simulink model "APF_SoftLanding_Quadrotor"  (R2023a)
settings: Solver=VariableStepAuto  StartTime=0.0  StopTime=120  RelTol=1e-3
values from neighbouring files (symbols this model uses):
  alpha_t = pi/2    (= 1.57079632679)    [Parameters.m]
  d0 = 7    [Parameters.m]
  k1 = 0.1395    [Parameters.m]
  k2 = 0.1784    [Parameters.m]
  k3 = 0.0442    [Parameters.m]
  ka = 0.2    [Parameters.m]
  katt = 10    [Parameters.m]
  kb = 0.6    [Parameters.m]
  kc = 0.4    [Parameters.m]
  krep = 90000    [Parameters.m]
  m = 5    [Parameters.m]
  maxRange = 10    [Parameters.m]
  n = 3    [Parameters.m]
  P_psi_lead = 2    [Parameters.m]
  P_vel_lead = 5    [Parameters.m]
  posHpad = [-25 -25 0]    [Parameters.m]
  Rmin = 0.1    [Parameters.m]
  target = [-25 -25 -5]    [Parameters.m]
  theta_des = pi/4    (= 0.785398163397)    [Parameters.m]
  thresholdLanding = 15    [Parameters.m]
  v_max = 2    [Parameters.m]
  zeta_des = 0    [Parameters.m]
  zGround = -0.15    [Parameters.m]
undefined symbols (not defined in the file or in its folder): Lidar, numobs, obs, platformUAV
libraries: uavsimlib x5, sharedtransform x2, uavalgslib x1, uavutilslib x1
(part 1 of 3)

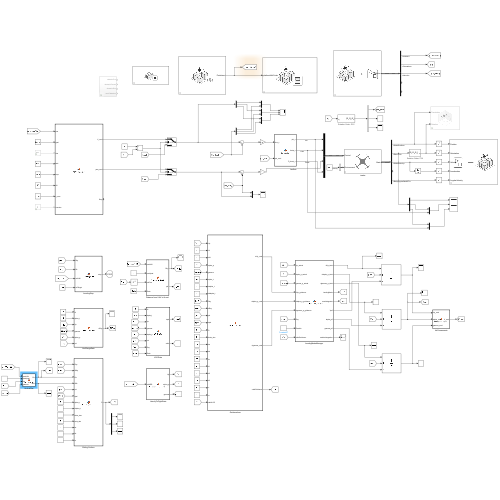
[thumbnail: Simulink's stored preview of the top-level diagram]
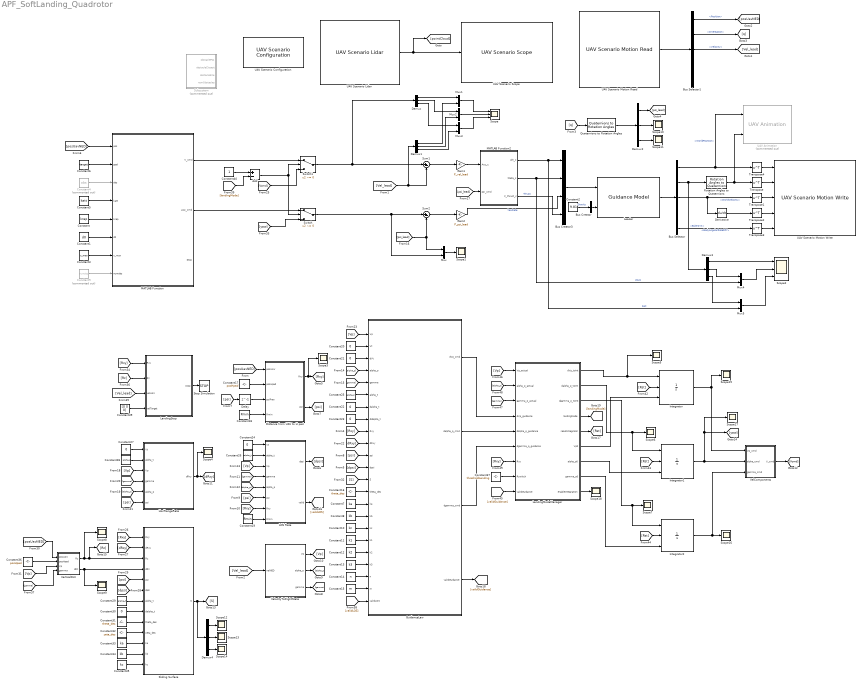
== system APF_SoftLanding_Quadrotor ==
  Add : Sum  Inputs=+-
  Bus Creator : BusCreator  Inputs=1  OutDataTypeStr=Bus: MultirotorGuidanceEnvironmentBus  NonVirtualBus=on
  Bus Creator3 : BusCreator  Inputs=4  OutDataTypeStr=Bus: MultirotorGuidanceControlBus  NonVirtualBus=on
  Bus Selector : BusSelector  OutputSignals=WorldPosition,EulerZYX,WorldVelocity,Thrust,BodyAngularRateRPY
  Bus Selector1 : BusSelector  OutputSignals=Position,Orientation,Velocity,Acceleration,AngularVelocity
  Constant : Constant  Value=krep
  Constant1 : Constant  Value=d0
  Constant10 : Constant  Value=kc
  Constant11 : Constant  Value=k1
  Constant12 : Constant  Value=k2
  Constant13 : Constant  Value=k3
  Constant14 : Constant  Value=n
  Constant15 : Constant  Value=m
  Constant16 : Constant  Value=theta_des
  Constant17 : Constant  Value=posHpad
  Constant18 : Constant  Value=Rmin
  Constant19 : Constant  Value=Rmin
  Constant2 : Constant  Value=9.81
  Constant{20..24,27,30} (7 alike) : Constant  Value=0
  Constant{25..26,28..29} (4 alike) : Constant  Value=alpha_t
  Constant3 : Constant  Value=v_max
  Constant31 : Constant  Value=theta_des
  Constant32 : Constant  Value=zeta_des
  Constant33 : Constant  Value=ka
  Constant34 : Constant  Value=kb
  Constant35 : Constant  Value=kc
  Constant36 : Constant  Value=posHpad
  Constant37 : Constant  Value=thresholdLanding
  Constant39 : Constant  Value=[0 0 0]
  Constant4 : Constant  Commented=on  Value=obs  VectorParams1D=off
  Constant40 : Constant
  Constant5 : Constant  Value=katt
  Constant6 : Constant  Value=target
  Constant7 : Constant  Value=ka
  Constant8 : Constant  Value=kb
  Constant9 : Constant  Commented=on  Value=numobs
  Delay : Delay  DelayLength=1
  Demux{,1..4} (5 alike) : Demux  Outputs=3
  Derivative : Derivative
  "Distance from UAV to H pad " : MATLAB Function  TreatAsAtomicUnit=on
  Gain1 : Gain  Gain=P_vel_lead
  Gain2 : Gain  Gain=P_psi_lead
  GuidanceLaw : MATLAB Function  TreatAsAtomicUnit=on
  HoriRangeRate : MATLAB Function  TreatAsAtomicUnit=on
  Integrator : Integrator  ExternalReset=rising  InitialConditionSource=external  InitialCondition=0.001
  Integrator1 : Integrator  ExternalReset=rising  InitialConditionSource=external
  Integrator2 : Integrator  ExternalReset=rising  InitialConditionSource=external
  LOS Rate : MATLAB Function  TreatAsAtomicUnit=on
  LandingModeManager : MATLAB Function  TreatAsAtomicUnit=on
  LandingStop : MATLAB Function  TreatAsAtomicUnit=on
  Leader : uavalgslib/Guidance Model  ModelType=MultirotorGuidance  SpecifiedDataType=double  SimulateUsing=Interpreted execution  InitialWorldPositionMultirotor=[-50; -50; -5]  InitialWorldVelocityMultirotor=[0.01; 0.01; 0.01]  InitialEulerZYXMultirotor=[0; 0; 0]  InitialBodyAngularRateRPYMultirotor=[0; 0; 0]  InitialThrustMultirotor=0  InitialNorthFixedWing=0  InitialEastFixedWing=0  InitialHeightFixedWing=0  InitialAirSpeedFixedWing=0  InitialHeadingAngleFixedWing=0  InitialFlightPathAngleFixedWing=0  InitialRollAngleFixedWing=0  InitialRollAngleRateFixedWing=0  PDRollMultirotor=[3402.97,116.67]  PDPitchMultirotor=[3402.97, 116.67]  PYawRateMultirotor=1950  PThrustMultirotor=3900  MassMultirotor=0.1  PHeightFixedWing=3.9  PHeadingAngleFixedWing=3.9  PFlightPathAngleFixedWing=39  PDRollFixedWing=[3402.97, 116.67]  PAirSpeedFixedWing=1  FlightPathAngleLimitsFixedWing=[-pi/2, pi/2]  StateBusName='MultirotorGuidanceStateBus'  ControlBusName='MultirotorGuidanceControlBus'  EnvironmentBusName='MultirotorGuidanceEnvironmentBus'  DataType=double
  MATLAB Function : MATLAB Function  TreatAsAtomicUnit=on
  MATLAB Function2 : MATLAB Function  TreatAsAtomicUnit=on
  Mux{,1..5} (6 alike) : Mux  Inputs=2
  Quaternions to Rotation Angles : sharedtransform/Quaternions to Rotation Angles  rotationOrder=ZYX  aMode=aMode
  Rotation Angles to Quaternions : sharedtransform/Rotation Angles to Quaternions  rotationOrder=ZYX  aMode=aMode
  Scope : Scope  NumInputPorts=3
  Scope{1,3..18} (17 alike) : Scope
  Scope2 : Scope  NumInputPorts=3
  Sliding Surface : MATLAB Function  TreatAsAtomicUnit=on
  Stop Simulation : Stop
  Subsystem : Subsystem  Commented=on
  Sum1 : Sum  Inputs=|+-
  Sum2 : Sum  Inputs=|+-
  Switch : Switch  Criteria=u2 ~= 0  Threshold=thresholdLanding  SaturateOnIntegerOverflow=off  InputSameDT=off
  Switch1 : Switch  Criteria=u2 ~= 0  Threshold=thresholdLanding  SaturateOnIntegerOverflow=off  InputSameDT=off
  Transpose{,1..4} (5 alike) : Math  Operator=transpose
  UAV Animation : uavutilslib/UAV Animation  Commented=on  UAVType=Multirotor  UAVSize=1  InertialZDirection=Down  SampleTime=-1
  UAV Scenario Configuration : uavsimlib/UAV Scenario Configuration  Priority=-1  UAVScenarioObject=sceneUAV  SampleTime=0.1  UpdateParam=false  SensorMotionBusName='SensorMotionBus'  PlatformMotionBusName='PlatformMotionBus'  ScenarioMotionBusName='ScenarioMotionBus'  ScenarioMotionSignalName='ScenarioMotions'
  UAV Scenario Lidar : uavsimlib/UAV Scenario Lidar  Priority=1  SensorName=platformUAV/Lidar  MaxRange=10  RangeAccuracy=0.002  AzimuthLimits=[ -43.5, 43.5 ]  AzimuthResolution=0.16  ElevationLimits=[ -29, 29 ]  ElevationResolution=1.25  HasNoise=on  HasOrganizedOutput=off  SampleTime=0.1
  UAV Scenario Motion Read : uavsimlib/UAV Scenario Motion Read  Priority=1  EntityName='platformUAV'  ReferenceFrame=NED
  UAV Scenario Motion Write : uavsimlib/UAV Scenario Motion Write  Priority=0  PlatName='platformUAV'  ReferenceFrame=NED
  UAV Scenario Scope : uavsimlib/UAV Scenario Scope  Priority=1  SensorNameTable={ 'platformUAV/Lidar', 'on' }  SampleTime=0.1
  VelComponents : MATLAB Function  TreatAsAtomicUnit=on
  VelocityToFlightState : MATLAB Function  TreatAsAtomicUnit=on
  VerticalDist : MATLAB Function  TreatAsAtomicUnit=on
  wires:
  Bus Creator/1 -> Leader/2
  Constant2/1 -> Bus Creator/1  "Gravity"
  Leader/1 -> Bus Selector/1
  Demux2/1 -> [psi_lead]
  Gain1/1 -> MATLAB Function2/1(Acc_c)
  Bus Creator3/1 -> Leader/1
  MATLAB Function2/1(phi_c) -> Mux5/2, Bus Creator3/1  "Roll"
  MATLAB Function2/2(theta_c) -> Mux4/2, Bus Creator3/2  "Pitch"
  Sum1/1 -> Gain1/1
  Sum2/1 -> Gain2/1
  [psi_lead] -> MATLAB Function2/2(psi_cmd)
  Gain2/1 -> Bus Creator3/3  "YawRate"
  MATLAB Function2/3(F_thrust_c) -> Bus Creator3/4  "Thrust"
  Bus Selector/1 -> Transpose4/1, UAV Animation/1  "<WorldPosition>"
  [Vel_lead] -> Demux1/1, Sum1/2
  UAV Scenario Lidar/1 -> [pointCloud], UAV Scenario Scope/1
  Bus Selector/2 -> Rotation Angles to Quaternions/1, Demux3/1  "<EulerZYX>"
  Rotation Angles to Quaternions/1 -> Transpose/1, UAV Animation/2
  Bus Selector/3 -> Transpose1/1, Derivative/1  "<WorldVelocity>"
  UAV Scenario Motion Read/1 -> Bus Selector1/1
  Quaternions to Rotation Angles/1 -> Demux2/1
  Bus Selector1/3 -> [Vel_lead]  "<Velocity>"
  Bus Selector1/1 -> [posUavNED]  "<Position>"
  Bus Selector1/2 -> [q]  "<Orientation>"
  [q] -> Quaternions to Rotation Angles/1
  [posUavNED] -> MATLAB Function/1(pos)
  Transpose4/1 -> UAV Scenario Motion Write/1
  Transpose/1 -> UAV Scenario Motion Write/2
  Transpose1/1 -> UAV Scenario Motion Write/3
  Derivative/1 -> Transpose2/1
  Transpose2/1 -> UAV Scenario Motion Write/4
  Bus Selector/5 -> Transpose3/1  "<BodyAngularRateRPY>"
  Transpose3/1 -> UAV Scenario Motion Write/5
  Mux/1 -> Scope1/1
  [psi_lead] -> Mux/1, Sum2/2
  Mux1/1 -> Scope/1
  Demux/1 -> Mux1/1
  Demux1/1 -> Mux1/2
  Mux2/1 -> Scope/2
  Demux/2 -> Mux2/1
  Demux1/2 -> Mux2/2
  Mux3/1 -> Scope/3
  Demux1/3 -> Mux3/2
  Demux/3 -> Mux3/1
  Constant4/1 -> MATLAB Function/3(obs)
  Constant9/1 -> MATLAB Function/8(numobs)
  Demux3/1 -> Scope2/1
  Mux4/1 -> Scope2/2
  Demux3/2 -> Mux4/1
  Mux5/1 -> Scope2/3
  Demux3/3 -> Mux5/1
  Constant5/1 -> MATLAB Function/4(katt)
  Constant/1 -> MATLAB Function/5(krep)
  Constant1/1 -> MATLAB Function/6(d0)
  Constant3/1 -> MATLAB Function/7(v_max)
  Constant11/1 -> GuidanceLaw/18(k1)
  Constant13/1 -> GuidanceLaw/20(k3)
  Constant14/1 -> GuidanceLaw/21(n)
  Constant15/1 -> GuidanceLaw/22(m)
  Constant7/1 -> GuidanceLaw/15(ka)
  Constant8/1 -> GuidanceLaw/16(kb)
  Constant10/1 -> GuidanceLaw/17(kc)
  Constant12/1 -> GuidanceLaw/19(k2)
  Constant16/1 -> GuidanceLaw/14(theta_des)
  Constant17/1 -> "Distance from UAV to H pad "/2(posHpad)
  [posUavNED] -> "Distance from UAV to H pad "/1(posUAV)
  Delay/1 -> "Distance from UAV to H pad "/3(psiPrev)
  "Distance from UAV to H pad "/1(Rxy) -> Scope3/1, [Rxy]
  [Rxy] -> GuidanceLaw/9(Rxy)
  Constant18/1 -> "Distance from UAV to H pad "/4(Rmin)
  Constant19/1 -> LOS Rate/8(Rmin)
  Constant20/1 -> GuidanceLaw/2(Vt)
  Constant21/1 -> GuidanceLaw/3(dVt)
  Constant23/1 -> GuidanceLaw/8(ddalpha_t)
  Constant22/1 -> GuidanceLaw/7(dalpha_t)
  [Vel_lead] -> VelocityToFlightState/1(velNED)
  LOS Rate/1(dpsi) -> [dpsi]
  [dpsi] -> GuidanceLaw/12(dpsi)
  "Distance from UAV to H pad "/2(psi) -> [psi]
  [psi] -> Delay/1
  [psi] -> GuidanceLaw/11(psi)
  [psi] -> LOS Rate/6(psi)
  [Rxy] -> LOS Rate/7(Rxy)
  Constant24/1 -> LOS Rate/1(Vt)
  Constant25/1 -> GuidanceLaw/6(alpha_t)
  VelocityToFlightState/3(gamma) -> [gamma]
  [gamma] -> LOS Rate/4(gamma)
  VelocityToFlightState/2(alpha_p) -> [alpha_p]
  [alpha_p] -> LOS Rate/5(alpha_p)
  VelocityToFlightState/1(Vp) -> [Vp]
  [Vp] -> LOS Rate/3(Vp)
  Constant26/1 -> LOS Rate/2(alpha_t)
  [alpha_p] -> GuidanceLaw/4(alpha_p)
  [gamma] -> GuidanceLaw/5(gamma)
  HoriRangeRate/1(dRxy) -> Scope4/1, [dRxy]
  [Vp] -> HoriRangeRate/3(Vp)
  [alpha_p] -> HoriRangeRate/5(alpha_p)
  [gamma] -> HoriRangeRate/4(gamma)
  [psi] -> HoriRangeRate/6(psi)
  [dRxy] -> GuidanceLaw/10(dRxy)
  Constant6/1 -> MATLAB Function/2(goal)
  Switch1/1 -> Demux/1, Sum1/1
  MATLAB Function/1(V_cmd) -> Switch1/1
  Switch/1 -> Mux/2, Sum2/1
  MATLAB Function/2(yaw_cmd) -> Switch/1
  GuidanceLaw/1(dVp_cmd) -> LandingModeManager/4(dVp_guidance)
  GuidanceLaw/2(dalpha_p_cmd) -> LandingModeManager/5(dalpha_p_guidance)
  GuidanceLaw/3(dgamma_cmd) -> LandingModeManager/6(dgamma_p_guidance)
  [Vp] -> GuidanceLaw/1(Vp)
  Constant27/1 -> HoriRangeRate/1(Vt)
  Constant28/1 -> HoriRangeRate/2(alpha_t)
  Sliding Surface/1(S) -> Demux4/1, [S]
  [Rxy] -> Sliding Surface/1(Rxy)
  [dRxy] -> Sliding Surface/2(dRxy)
  [psi] -> Sliding Surface/5(psi)
  [dpsi] -> Sliding Surface/6(dpsi)
  VerticalDist/2(dRz) -> Scope9/1, Sliding Surface/4(dRz)
  VerticalDist/1(Rz) -> Sliding Surface/3(Rz), [Rz], Scope8/1
  [posUavNED] -> VerticalDist/1(posUAV)
  Constant29/1 -> Sliding Surface/7(alpha_t)
  Constant30/1 -> Sliding Surface/8(dalpha_t)
  Constant31/1 -> Sliding Surface/9(theta_des)
  Constant32/1 -> Sliding Surface/10(zeta_des)
  Constant34/1 -> Sliding Surface/12(kb)
  Constant33/1 -> Sliding Surface/11(ka)
  Constant35/1 -> Sliding Surface/13(kc)
  Constant36/1 -> VerticalDist/2(posHpad)
  [S] -> GuidanceLaw/13(S)
  [Vcmd] -> Switch1/3
  [yaw] -> Switch/3
  LandingStop/1(stop) -> Stop Simulation/1
  [Rxy] -> LandingStop/1(Rxy)
  [Rz] -> LandingStop/2(Rz)
  [Vel_lead] -> LandingStop/3(velUAV)
  Constant39/1 -> LandingStop/4(velTarget)
  [Vp] -> VerticalDist/3(Vp)
  [gamma] -> VerticalDist/4(gamma)
  Demux2/2 -> Scope10/1
  Demux2/3 -> Scope11/1
  Demux4/1 -> Scope12/1
  Demux4/2 -> Scope13/1
  Demux4/3 -> Scope14/1
  LOS Rate/2(valid) -> [validLOS]
  [validLOS] -> GuidanceLaw/23(validLOS)
  GuidanceLaw/4(validGuidance) -> [validGuidance]
  [validGuidance] -> LandingModeManager/9(validGuidance)
  [Rst] -> Integrator1/2
  [Rst] -> Integrator/2
  [Rst] -> Integrator2/2
  LandingModeManager/1(dVp_toInt) -> Scope5/1, Integrator/1
  Integrator/1 -> Scope15/1, VelComponents/1(Vp_cmd)
  Integrator1/1 -> Scope17/1, [yaw], VelComponents/2(alpha_cmd)
  VelComponents/1(V_cmd) -> [Vcmd]
  Integrator2/1 -> VelComponents/3(gamma_cmd), Scope16/1
  LandingModeManager/2(dalpha_p_toInt) -> Integrator1/1, Scope6/1
  LandingModeManager/3(dgamma_p_toInt) -> Integrator2/1, Scope7/1
  LandingModeManager/5(resetIntegrator) -> [Rst]
  [Vp] -> LandingModeManager/1(Vp_actual)
  [gamma] -> LandingModeManager/3(gamma_p_actual)
  [alpha_p] -> LandingModeManager/2(alpha_p_actual)
  [Rxy] -> LandingModeManager/7(Rxy)
  Constant37/1 -> LandingModeManager/8(Rswitch)
  LandingModeManager/6(Vp0) -> Integrator/3
  LandingModeManager/7(alpha_p0) -> Integrator1/3
  LandingModeManager/8(gamma_p0) -> Integrator2/3
  LandingModeManager/9(enableIntegration) -> Scope18/1
  LandingModeManager/4(landingMode) -> [landingMode]
  [landingMode] -> Add/2
  Add/1 -> Switch1/2, Switch/2
  Constant40/1 -> Add/1

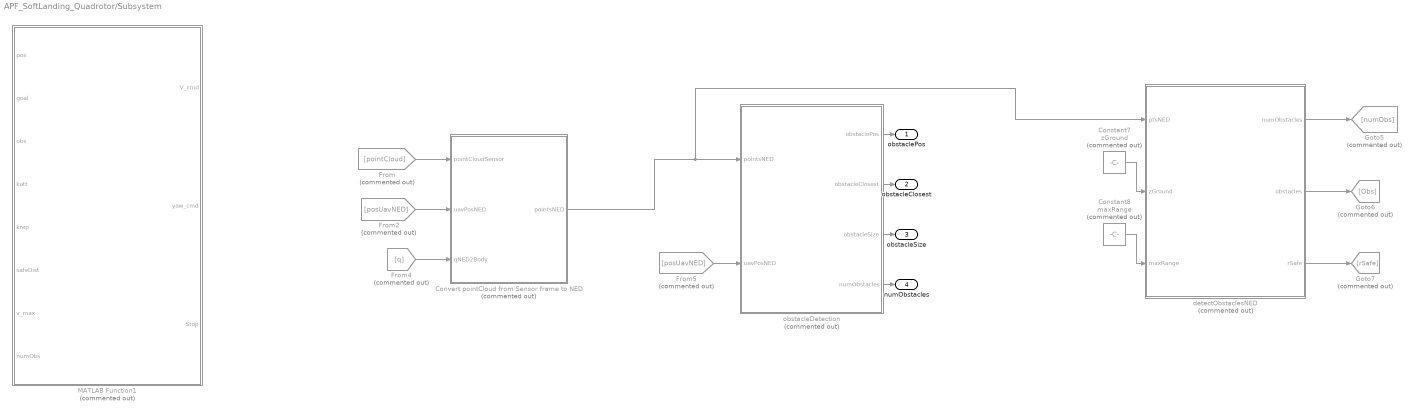
== system APF_SoftLanding_Quadrotor/Subsystem ==
  Constant7 : Constant  Commented=on  Value=zGround
  Constant8 : Constant  Commented=on  Value=maxRange
  Convert pointCloud from Sensor frame to NED : MATLAB Function  Commented=on  TreatAsAtomicUnit=on
  From : From  Commented=on  GotoTag=pointCloud
  From2 : From  Commented=on  GotoTag=posUavNED
  From4 : From  Commented=on  GotoTag=q
  From5 : From  Commented=on  GotoTag=posUavNED
  Goto5 : Goto  Commented=on  GotoTag=numObs
  Goto6 : Goto  Commented=on  GotoTag=Obs
  Goto7 : Goto  Commented=on  GotoTag=rSafe
  MATLAB Function1 : MATLAB Function  Commented=on  TreatAsAtomicUnit=on
  detectObstaclesNED : MATLAB Function  Commented=on  TreatAsAtomicUnit=on
  obstacleDetection : MATLAB Function  Commented=on  TreatAsAtomicUnit=on
  obstaclePos : Outport
  obstacleClosest : Outport  Port=2
  obstacleSize : Outport  Port=3
  numObstacles : Outport  Port=4
  wires:
  From4/1 -> Convert pointCloud from Sensor frame to NED/3(qNED2Body)
  Convert pointCloud from Sensor frame to NED/1(pointsNED) -> detectObstaclesNED/1(ptsNED), obstacleDetection/1(pointsNED)
  From2/1 -> Convert pointCloud from Sensor frame to NED/2(uavPosNED)
  detectObstaclesNED/1(numObstacles) -> Goto5/1
  obstacleDetection/1(obstaclePos) -> obstaclePos/1
  From/1 -> Convert pointCloud from Sensor frame to NED/1(pointCloudSensor)
  detectObstaclesNED/2(obstacles) -> Goto6/1
  Constant8/1 -> detectObstaclesNED/3(maxRange)
  Constant7/1 -> detectObstaclesNED/2(zGround)
  detectObstaclesNED/3(rSafe) -> Goto7/1
  From5/1 -> obstacleDetection/2(uavPosNED)
  obstacleDetection/3(obstacleSize) -> obstacleSize/1
  obstacleDetection/2(obstacleClosest) -> obstacleClosest/1
  obstacleDetection/4(numObstacles) -> numObstacles/1

== matlab function APF_SoftLanding_Quadrotor/MATLAB Function2 ==
function [phi_c, theta_c, F_thrust_c] = Conversion(Acc_c, psi_cmd)

% =========================================================
% Nonlinear acceleration -> attitude/thrust conversion
% Coordinate frame: NED
%
% Acc_c   = [aN; aE; aD] [m/s^2]
% psi_cmd = desired yaw  [rad]
% =========================================================

g = 9.81;
m = 0.1;     % kg

aN = Acc_c(1);
aE = Acc_c(2);
aD = Acc_c(3);

psi = psi_cmd;

% ---------------------------------------------------------
% Required thrust vector
%
% m*a = m*g*e3 - T*b3
%
% Therefore:
%
% T*b3 = m*[ -aN, -aE, g-aD ]
% ---------------------------------------------------------

fN = -aN;
fE = -aE;
fD =  g - aD;

f_norm = sqrt(fN^2 + fE^2 + fD^2);

if f_norm > 1e-6

    % Desired body-Z direction
    b3N = fN / f_norm;
    b3E = fE / f_norm;
    b3D = fD / f_norm;

    % -----------------------------------------------------
    % Desired roll
    % -----------------------------------------------------

    sin_phi = sin(psi)*b3N - cos(psi)*b3E;

    % Numerical protection
    sin_phi = max(min(sin_phi,1.0),-1.0);

    phi_c = asin(sin_phi);

    % -----------------------------------------------------
    % Desired pitch
    % -----------------------------------------------------

    theta_c = atan2( ...
        cos(psi)*b3N + sin(psi)*b3E, ...
        b3D);

    % -----------------------------------------------------
    % Thrust magnitude
    % -----------------------------------------------------

    F_thrust_c = m*f_norm;

else

    phi_c = 0.0;
    theta_c = 0.0;
    F_thrust_c = 0.0;

end

% ---------------------------------------------------------
% Safety limits
% ---------------------------------------------------------

phi_max   = pi/4;
theta_max = pi/4;

phi_c = max(min(phi_c, phi_max), -phi_max);
theta_c = max(min(theta_c, theta_max), -theta_max);

F_thrust_c = max(F_thrust_c,0.0);

end
%%=========================================================================

% function [phi_c, theta_c, F_thrust_c] = Conversion(Acc_c, psi_lead)
%     % Acc_c: Vector gia tốc mong muốn [ax; ay; az] từ bộ điều khiển P
%     % psi: Góc Yaw hiện tại (rad)
%     % m: Khối lượng UAV (kg)
% 
%     % Hằng số trọng trường
%     g = 9.81;
% 
%     % Trích xuất các thành phần gia tốc
%     ax = Acc_c(1);
%     ay = Acc_c(2);
%     az = Acc_c(3);
% 
%     % 1. Tính góc Roll lệnh (phi_c)
%     phi_c = (1/g) * (ay * cos(psi_lead) - ax * sin(psi_lead));
% 
%     % 2. Tính góc Pitch lệnh (theta_c)
%     theta_c = -(1/g) * (ax * cos(psi_lead) + ay * sin(psi_lead));
% 
%     % 3. Tính lực đẩy lệnh (F_thrust_c)
%     % Công thức trong hệ NED: m * (g - az)
%     % Lưu ý: Trong hệ NED, gia tốc az âm là hướng lên, dương là hướng xuống.
%     F_thrust_c = 0.1 * (g - az);
% 
%     % Giới hạn giá trị (Safety Clamp) để tránh máy bay bị crash khi lệnh quá lớn
%     phi_c = max(min(phi_c, deg2rad(45)), deg2rad(-45));
%     theta_c = max(min(theta_c, deg2rad(45)), deg2rad(-45));
% end

== matlab function APF_SoftLanding_Quadrotor/Distance from UAV to H pad  ==
function [Rxy, psi] = DistUAVtoHpad(posUAV, posHpad, psiPrev, Rmin)
dx = posHpad(1) - posUAV(1);
dy = posHpad(2) - posUAV(2);

Rxy2 = dx*dx + dy*dy;
Rxy  = sqrt(Rxy2);

valid = Rxy > Rmin;

if valid
    psi  = atan2(dy, dx);
else
    psi  = psiPrev;
end
end

== matlab function APF_SoftLanding_Quadrotor/LOS Rate ==
function [dpsi, valid] = LOSRate( ...
    Vt, alpha_t, Vp, gamma, alpha_p, psi, Rxy, Rmin)

% Speeds: m/s; distances: m
% Angles: rad; dpsi: rad/s
% Rmin must be positive.

valid = (Rxy > Rmin) && (Rmin > 0);

if valid
    % Equation (4)
    dpsi = (Vt*sin(alpha_t - psi) ...
          - Vp*cos(gamma)*sin(alpha_p - psi)) / Rxy;
else
    % Numerical fallback, not the actual LOS angular rate.
    dpsi = 0;
end
end

== matlab function APF_SoftLanding_Quadrotor/VelocityToFlightState ==
function [Vp, alpha_p, gamma] = VelocityToFlightState(velNED)
% velNED: WorldVelocity, vector 3x1, m/s
% alpha_p and gamma: rad
% gamma positive upward, following the paper

vx = velNED(1);
vy = velNED(2);
vz = velNED(3);

Vxy = hypot(vx, vy);

Vp      = sqrt(vx*vx + vy*vy + vz*vz);
alpha_p = atan2(vy, vx);
gamma   = atan2(-vz, Vxy);
end

== matlab function APF_SoftLanding_Quadrotor/HoriRangeRate ==
function dRxy = HoriRangeRate(Vt, alpha_t, Vp, gamma, alpha_p, psi)
% Vt, Vp: m/s
% All angles: rad
% dRxy: m/s

dRxy = Vt*cos(alpha_t - psi) ...
     - Vp*cos(gamma)*cos(alpha_p - psi);

end

== matlab function APF_SoftLanding_Quadrotor/VelComponents ==
function V_cmd  = VelComponents(Vp_cmd, alpha_cmd, gamma_cmd)
% Vp: m/s
% gamma, alpha_p: rad
% Outputs: velocity in NED, m/s

Vx =  Vp_cmd*cos(gamma_cmd)*cos(alpha_cmd);
Vy =  Vp_cmd*cos(gamma_cmd)*sin(alpha_cmd);
Vz =  -Vp_cmd*sin(gamma_cmd);

V_cmd = [Vx Vy Vz];
end

== matlab function APF_SoftLanding_Quadrotor/Sliding Surface ==
function S = SlidingSurface(Rxy, dRxy, Rz, dRz, ...
    psi, dpsi, alpha_t, dalpha_t, ...
    theta_des, zeta_des, ka, kb, kc)
% Distances: m; range rates: m/s
% Angles: rad; angular rates: rad/s
% S: 3x1 vector
%
% psi: LOS azimuth, not UAV body yaw
% theta_des: desired LOS elevation
% zeta_des: desired LOS azimuth relative to target heading

% Equation (17): horizontal range
S1 = dRxy + ka*Rxy;

% Equation (17): vertical range and elevation constraint
td = tan(theta_des);

S2 = dRz + td*dRxy ...
   + kb*(Rz + td*Rxy);

% Equation (17): relative azimuth constraint
%e_psi = psi - alpha_t - zeta_des;
e_raw = psi - alpha_t - zeta_des;
e_psi = atan2(sin(e_raw), cos(e_raw));
S3 = (dpsi - dalpha_t) + kc*e_psi;

% Input to guidanceLaw
S = [S1; S2; S3];

end

== matlab function APF_SoftLanding_Quadrotor/VerticalDist ==
function [Rz, dRz] = VerticalDist(posUAV, posHpad, Vp, gamma)
%Rz  =  posHpad(3) - posUAV(3);
Rz  =  posUAV(3) - posHpad(3);
dRz =  -Vp * sin(gamma);
end

== matlab function APF_SoftLanding_Quadrotor/LandingStop ==
function stop = LandingStop(Rxy, Rz, velUAV, velTarget)
% velUAV and velTarget must use the same coordinate frame
% and have matching dimensions.
stop = 0;
dv = velUAV - velTarget;
vRel = sqrt(dv(1)^2 + dv(2)^2 + dv(3)^2);

% stop = (Rxy <= 0.1) ...
%     && (abs(Rz) <= 0.1) ...
%     && (vRel <= vTol);
if (Rxy <= 0.1) || (abs(Rz) <= 0.1)
    stop = 1;
end
end

== matlab function APF_SoftLanding_Quadrotor/LandingModeManager ==
function [dVp_toInt, dalpha_p_toInt, dgamma_p_toInt, ...
          landingMode, resetIntegrator, ...
          Vp0, alpha_p0, gamma_p0, enableIntegration] = ...
    LandingModeManager( ...
    Vp_actual, alpha_p_actual, gamma_p_actual, ...
    dVp_guidance, dalpha_p_guidance, dgamma_p_guidance, ...
    Rxy, Rswitch, validGuidance)

% All inputs scalar; validGuidance logical.
% Actual states come from measured UAV velocity, NOT Landing Integrators.
% Units: speed [m/s], angles [rad], distance [m].
% gamma_p_actual is positive upward.
% GuidanceLaw must run in APF as well to evaluate readiness for handover.
%
% landingMode: false = APF; true = Landing, latched for this simulation.
% resetIntegrator: one-sample pulse only on APF -> Landing.
% x0 outputs follow valid actual states in APF, then freeze at handover.
% d*_toInt: guidance derivatives when enabled, otherwise zero.

persistent inLanding VpInit alphaInit gammaInit
if isempty(inLanding)
    inLanding = false;
    VpInit = 0;
    alphaInit = 0;
    gammaInit = 0;
end

resetIntegrator = false;
dVp_toInt = 0;
dalpha_p_toInt = 0;
dgamma_p_toInt = 0;

stateOK = isfinite(Vp_actual) && Vp_actual > 1e-6 ...
    && isfinite(alpha_p_actual) && isfinite(gamma_p_actual) ...
    && abs(cos(gamma_p_actual)) > 1e-6;

ratesOK = isfinite(dVp_guidance) ...
    && isfinite(dalpha_p_guidance) && isfinite(dgamma_p_guidance);

distanceOK = isfinite(Rxy) && Rxy > 0;
guidanceOK = validGuidance && stateOK && ratesOK && distanceOK;

rangeOK = distanceOK && isfinite(Rswitch) ...
    && Rswitch > 0 && Rxy <= Rswitch;

if ~inLanding
    % Use the actual UAV state at handover as the Landing initial state.
    if stateOK
        VpInit = Vp_actual;
        alphaInit = alpha_p_actual;
        gammaInit = gamma_p_actual;
    end

    if rangeOK && guidanceOK
        inLanding = true;
        resetIntegrator = true;
    end
end

% Pause integration on invalid guidance; keep Landing mode latched.
enableIntegration = inLanding && guidanceOK;
if enableIntegration
    dVp_toInt = dVp_guidance;
    dalpha_p_toInt = dalpha_p_guidance;
    dgamma_p_toInt = dgamma_p_guidance;
end

landingMode = inLanding;
Vp0 = VpInit;
alpha_p0 = alphaInit;
gamma_p0 = gammaInit;
end

== matlab function APF_SoftLanding_Quadrotor/Subsystem/Convert pointCloud from Sensor frame to NED ==
function pointsNED = pointCloudToNED(pointCloudSensor, uavPosNED, qNED2Body)
%#codegen
% Giới hạn cận trên cho biến variable-size (ví dụ tối đa 50000 điểm)
coder.varsize('pointsNED', [50000, 3], [1, 0]);
coder.varsize('pointCloudSensor', [50000, 3], [1, 0]);

%% 1. Kiểm tra đầu vào
if isempty(pointCloudSensor)
    pointsNED = zeros(0, 3);
    return;
end

% Đảm bảo định dạng ma trận Nx3
pointCloudSensor = reshape(pointCloudSensor, [], 3);

% Lọc bỏ NaN và Inf
valid = all(isfinite(pointCloudSensor), 2);
pointCloudSensor = pointCloudSensor(valid, :);

if isempty(pointCloudSensor)
    pointsNED = zeros(0, 3);
    return;
end

%% 2. Chuẩn hóa vị trí UAV (1x3)
uavPosNED = reshape(uavPosNED, 1, 3);

%% 3. Xử lý Quaternion và Ma trận xoay
q = reshape(qNED2Body, 1, 4);
qNorm = norm(q);
if qNorm > 1e-6
    q = q / qNorm;
else
    q = [1, 0, 0, 0]; % Tránh chia cho 0
end

% R_BN: chuyển từ NED -> Body
R_BN = quat2rotm(q);

% R_NB: chuyển từ Body -> NED (ma trận trực giao nên lấy chuyển vị)
R_NB = R_BN.';

%% 4. Chuyển đổi tọa độ sang hệ NED
% p_NED = p_Body * R_NB.' + p_UAV_NED (nhân ma trận trực tiếp nhanh hơn)
pointsNED = pointCloudSensor * R_BN + uavPosNED;

end
% function pointsNED = pointCloudToNED(pointCloudSensor, uavPosNED, qNED2Body)
% % pointCloudToNED
% % Convert LiDAR point cloud from Sensor/Body frame to NED frame.
% %
% % INPUT:
% %   pointCloudSensor : Nx3 point cloud [x y z] in sensor frame
% %   uavPosNED        : 1x3 or 3x1 UAV position [N E D]
% %   qNED2Body        : 1x4 quaternion [qw qx qy qz]
% %                      rotation from NED frame to UAV body frame
% %
% % OUTPUT:
% %   pointsNED        : Nx3 point cloud in NED frame
% %
% % ASSUMPTION:
% %   LiDAR is located at UAV body origin and aligned with body frame.
% 
%     %% Check input
%     if isempty(pointCloudSensor)
%         pointsNED = zeros(0,3);
%         return;
%     end
% 
%     % Make sure point cloud is Nx3
%     pointCloudSensor = reshape(pointCloudSensor, [], 3);
% 
%     % Remove NaN and Inf
%     valid = all(isfinite(pointCloudSensor), 2);   % isfinite(pointCloudSensor): Kiểm tra từng phần tử trong ma trận, all(..., 2): Kiểm tra theo chiều ngang( từng hàng)
%     pointCloudSensor = pointCloudSensor(valid, :);
% 
%     %% UAV position
%     uavPosNED = uavPosNED(:).';     % Force 1x3
% 
%     %% Normalize quaternion
%     qNED2Body = qNED2Body(:).';     % Đảm bảo vector có dạng 1x4
%     qNED2Body = qNED2Body / norm(qNED2Body);
% 
%     %% Rotation matrix
%     % R_BN: transforms NED coordinates -> Body coordinates
%     R_BN = quat2rotm(qNED2Body);
% 
%     % Therefore:
%     % R_NB = R_BN'
%     % transforms Body coordinates -> NED coordinates
%     R_NB = R_BN';
% 
%     %% Transform point cloud
%     %
%     % p_NED = R_NB * p_Body + p_UAV_NED
%     %
%     pointsNED = (R_NB * pointCloudSensor.').';
% 
%     pointsNED = pointsNED + uavPosNED;
% 
% end
